simulink model "proj4_BF"  (Simulink 5.0)
settings: Solver=ode45  StartTime=0.0  StopTime=10.0  RelTol=1e-3
settings Model: LastModifiedBy=Frank Gloria

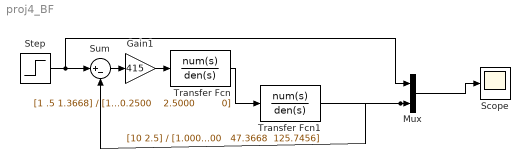
== system proj4_BF ==
  Gain1 : Gain  Gain=415  SaturateOnIntegerOverflow=on
  Mux : Mux  Inputs=2
  Scope : Scope
  Step : Step  Time=0  Before=1  SampleTime=0
  Sum : Sum  Inputs=|+-  SaturateOnIntegerOverflow=on
  Transfer Fcn : TransferFcn  Numerator=[1 .5 1.3668]  Denominator="[1.0000   10.2500    2.5000         0]"
  Transfer Fcn1 : TransferFcn  Numerator=[10 2.5]  Denominator="[1.0000   92.5000   47.3668  125.7456]"
  wires:
  Mux/1 -> Scope/1
  Transfer Fcn1/1 -> Sum/2, Mux/2
  Step/1 -> Sum/1, Mux/1
  Sum/1 -> Gain1/1
  Gain1/1 -> Transfer Fcn/1
  Transfer Fcn/1 -> Transfer Fcn1/1
